simulink model "im_kalman_xy"  (R2025a)
settings: Solver=daessc  StartTime=0.0  StopTime=simlength  MaxStep=Tc  RelTol=Tc
undefined symbols (not defined in the file): Ad, Bd, C, cp, Ibez, Im, Inom, J, ki_inv_d, kp_inv_d, Lm, Qkalman, Rkalman, start_load, Tc, Ts, Vdc, w0
libraries: nesl_utility x11, fl_lib x6, simulink x2, im_lib x1
settings Model: SimulationMode=accelerator  Creator=dbagn  LastModifiedBy=dbagn
settings SolverCC: AlgebraicLoopSolver=TrustRegion
settings DataIOCC: ReturnWorkspaceOutputs=off
settings DebuggingCC: UnconnectedInputMsg=warning  UnconnectedOutputMsg=warning  UnconnectedLineMsg=warning
settings ModelReferenceCC: EnableRefExpFcnMdlSchedulingChecks=on
settings RTWCC: GPUComputeCapability=3.5  DLArmComputeVersion=19.05

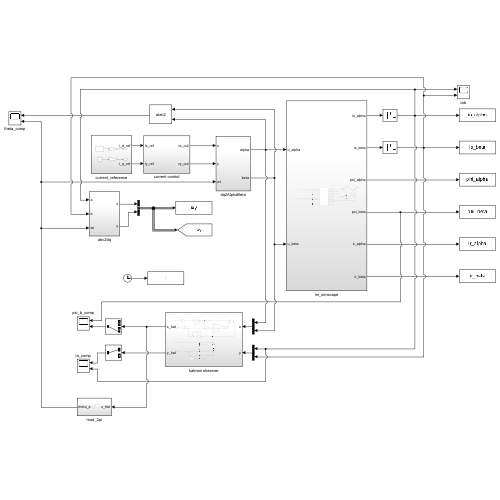
[thumbnail: Simulink's stored preview of the top-level diagram]
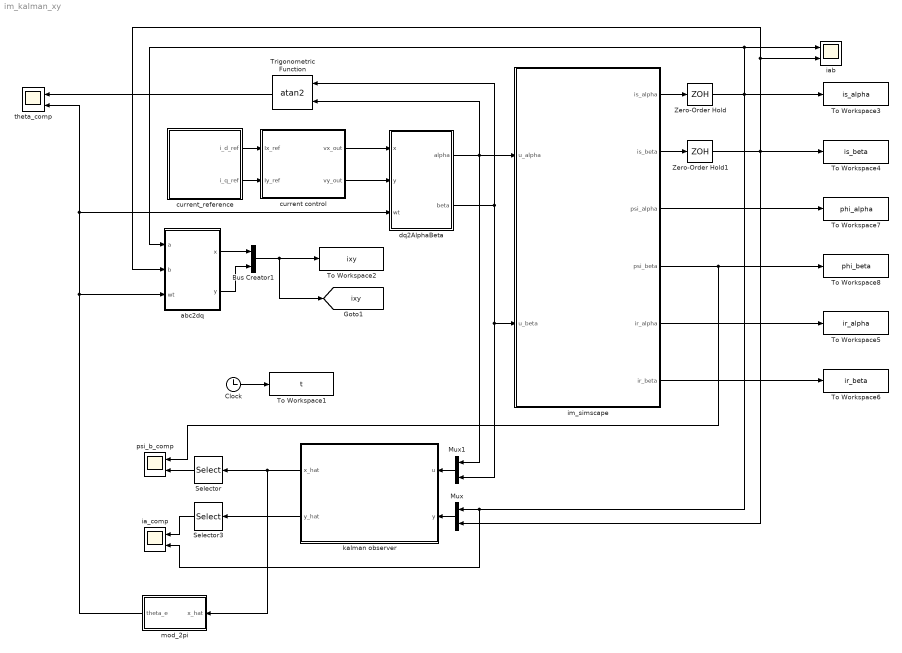
== system im_kalman_xy ==
  Bus Creator1 : BusCreator  Inputs=2
  Clock : Clock
  Mux : Mux  Inputs=2
  Mux1 : Mux  Inputs=2
  Selector : Selector  InputPortWidth=4  IndexOptions=Index vector (dialog)  Indices=4  OutputSizes=1
  Selector3 : Selector  InputPortWidth=2  IndexOptions=Index vector (dialog)  Indices=1  OutputSizes=1
  To Workspace1 : ToWorkspace  VariableName=t  SampleTime=Tc
      settings: MaxDataPoints=Nc
  To Workspace2 : ToWorkspace  VariableName=ixy  SampleTime=Tc
      settings: MaxDataPoints=Nc
  To Workspace3 : ToWorkspace  VariableName=is_alpha  SampleTime=Tc
      settings: MaxDataPoints=Nc
  To Workspace4 : ToWorkspace  VariableName=is_beta  SampleTime=Tc
      settings: MaxDataPoints=Nc
  To Workspace5 : ToWorkspace  VariableName=ir_alpha  SampleTime=Tc
      settings: MaxDataPoints=Nc
  To Workspace6 : ToWorkspace  VariableName=ir_beta  SampleTime=Tc
      settings: MaxDataPoints=Nc
  To Workspace7 : ToWorkspace  VariableName=phi_alpha  SampleTime=Tc
      settings: MaxDataPoints=Nc
  To Workspace8 : ToWorkspace  VariableName=phi_beta  SampleTime=Tc
      settings: MaxDataPoints=Nc
  Trigonometric Function : Trigonometry  Operator=atan2
  Zero-Order Hold : ZeroOrderHold  SampleTime=Ts
  Zero-Order Hold1 : ZeroOrderHold  SampleTime=Ts
  abc2dq : Subsystem
  current control : Subsystem
  current_reference : Subsystem
  dq2AlphaBeta : Subsystem
  ia_comp : Scope  NumInputPorts=2
      settings: ActiveDisplayYMinimum=-1099.3046905610083  ActiveDisplayYMaximum=2745.620661883479  DataLoggingVariableName=ScopeData3
  iab : Scope  NumInputPorts=2
      settings: ActiveDisplayYMinimum=-896.39173  ActiveDisplayYMaximum=667.17944
  im_simscape : Subsystem
  kalman observer : Subsystem
  mod_2pi : Subsystem
  psi_b_comp : Scope  NumInputPorts=2
      settings: ActiveDisplayYMinimum=-1.84097  ActiveDisplayYMaximum=1.77789  DataLoggingVariableName=ScopeData2
  theta_comp : Scope  NumInputPorts=2
      settings: ActiveDisplayYMinimum=-3.92689  ActiveDisplayYMaximum=3.92642
  tag scope: ixy=global
  wires:
  im_simscape/4(psi_beta) -> psi_b_comp/1, To Workspace8/1
  im_simscape/2(is_beta) -> Zero-Order Hold1/1
  im_simscape/1(is_alpha) -> Zero-Order Hold/1
  Mux1/1 -> kalman observer/1(u)
  Zero-Order Hold/1 -> Mux/1, ia_comp/2, To Workspace3/1, iab/1, abc2dq/1(a)
  Zero-Order Hold1/1 -> Mux/2, To Workspace4/1, abc2dq/2(b), iab/2
  Mux/1 -> kalman observer/2(y)
  Selector/1 -> psi_b_comp/2
  Selector3/1 -> ia_comp/1
  kalman observer/2(y_hat) -> Selector3/1
  current_reference/2(i_q_ref) -> current control/2(Iy_ref)
  current_reference/1(i_d_ref) -> current control/1(Ix_ref)
  Bus Creator1/1 -> To Workspace2/1, [ixy]
  abc2dq/2(y) -> Bus Creator1/2
  abc2dq/1(x) -> Bus Creator1/1
  current control/1(vx_out) -> dq2AlphaBeta/1(x)
  current control/2(vy_out) -> dq2AlphaBeta/2(y)
  dq2AlphaBeta/1(alpha) -> Trigonometric Function/2, Mux1/1, im_simscape/1(u_alpha)
  dq2AlphaBeta/2(beta) -> Mux1/2, im_simscape/2(u_beta), Trigonometric Function/1
  mod_2pi/1(theta_e) -> theta_comp/2, dq2AlphaBeta/3(wt), abc2dq/3(wt)
  Clock/1 -> To Workspace1/1
  kalman observer/1(x_hat) -> mod_2pi/1(x_hat), Selector/1
  im_simscape/3(psi_alpha) -> To Workspace7/1
  im_simscape/5(ir_alpha) -> To Workspace5/1
  im_simscape/6(ir_beta) -> To Workspace6/1
  Trigonometric Function/1 -> theta_comp/1

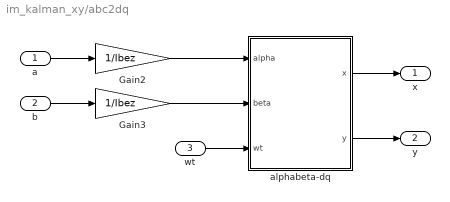
== system im_kalman_xy/abc2dq ==
  a : Inport
  b : Inport  Port=2
  wt : Inport  Port=3
  Gain2 : Gain  Gain=1/Ibez
  Gain3 : Gain  Gain=1/Ibez
  alphabeta-dq : Subsystem
  x : Outport  VectorParamsAs1DForOutWhenUnconnected=off
  y : Outport  Port=2  VectorParamsAs1DForOutWhenUnconnected=off
  wires:
  a/1 -> Gain2/1
  b/1 -> Gain3/1
  wt/1 -> alphabeta-dq/3(wt)
  alphabeta-dq/1(x) -> x/1
  alphabeta-dq/2(y) -> y/1
  Gain2/1 -> alphabeta-dq/1(alpha)
  Gain3/1 -> alphabeta-dq/2(beta)

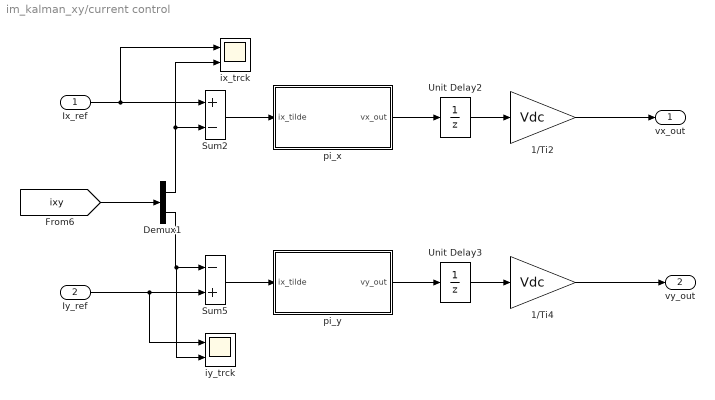
== system im_kalman_xy/current control ==
  Ix_ref : Inport
  Iy_ref : Inport  Port=2
  1/Ti2 : Gain  Gain=Vdc  SaturateOnIntegerOverflow=on  OutDataTypeStr=Inherit: Same as input  ParamDataTypeStr=Inherit: Same as input
  1/Ti4 : Gain  Gain=Vdc  SaturateOnIntegerOverflow=on  OutDataTypeStr=Inherit: Same as input  ParamDataTypeStr=Inherit: Same as input
  Demux1 : Demux  Outputs=2
  Sum2 : Sum  Inputs=+-  SaturateOnIntegerOverflow=on
  Sum5 : Sum  Inputs=-+  SaturateOnIntegerOverflow=on
  Unit Delay2 : UnitDelay  SampleTime=Ts  HasFrameUpgradeWarning=on
  Unit Delay3 : UnitDelay  SampleTime=Ts  HasFrameUpgradeWarning=on
  ix_trck : Scope  NumInputPorts=2
      settings: ActiveDisplayYMinimum=0.20638  ActiveDisplayYMaximum=0.72674
  iy_trck : Scope  NumInputPorts=2
      settings: ActiveDisplayYMinimum=-0.16299  ActiveDisplayYMaximum=1.1565  DataLoggingVariableName=ScopeData2
  pi_x : Subsystem
  pi_y : Subsystem
  vx_out : Outport  VectorParamsAs1DForOutWhenUnconnected=off
  vy_out : Outport  Port=2  VectorParamsAs1DForOutWhenUnconnected=off
  wires:
  Iy_ref/1 -> iy_trck/1, Sum5/2
  Unit Delay3/1 -> 1/Ti4/1
  Unit Delay2/1 -> 1/Ti2/1
  [ixy] -> Demux1/1
  Demux1/2 -> iy_trck/2, Sum5/1
  Ix_ref/1 -> ix_trck/1, Sum2/1
  Demux1/1 -> ix_trck/2, Sum2/2
  pi_x/1(vx_out) -> Unit Delay2/1
  pi_y/1(vy_out) -> Unit Delay3/1
  Sum5/1 -> pi_y/1(ix_tilde)
  Sum2/1 -> pi_x/1(ix_tilde)
  1/Ti2/1 -> vx_out/1
  1/Ti4/1 -> vy_out/1

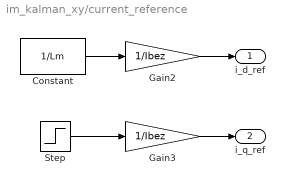
== system im_kalman_xy/current_reference ==
  Constant : Constant  Value=1/Lm
  Gain2 : Gain  Gain=1/Ibez
  Gain3 : Gain  Gain=1/Ibez
  Step : Step  Time=start_load  After=sqrt(Inom^2-Im^2)*sqrt(2)  SampleTime=0
  i_d_ref : Outport
  i_q_ref : Outport  Port=2
  wires:
  Step/1 -> Gain3/1
  Constant/1 -> Gain2/1
  Gain2/1 -> i_d_ref/1
  Gain3/1 -> i_q_ref/1

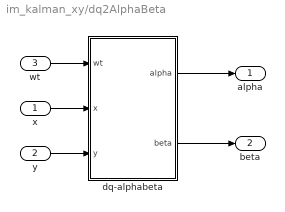
== system im_kalman_xy/dq2AlphaBeta ==
  x : Inport
  y : Inport  Port=2
  wt : Inport  Port=3
  dq-alphabeta : Subsystem
  alpha : Outport  VectorParamsAs1DForOutWhenUnconnected=off
  beta : Outport  Port=2  VectorParamsAs1DForOutWhenUnconnected=off
  wires:
  x/1 -> dq-alphabeta/2(x)
  y/1 -> dq-alphabeta/3(y)
  wt/1 -> dq-alphabeta/1(wt)
  dq-alphabeta/1(alpha) -> alpha/1
  dq-alphabeta/2(beta) -> beta/1

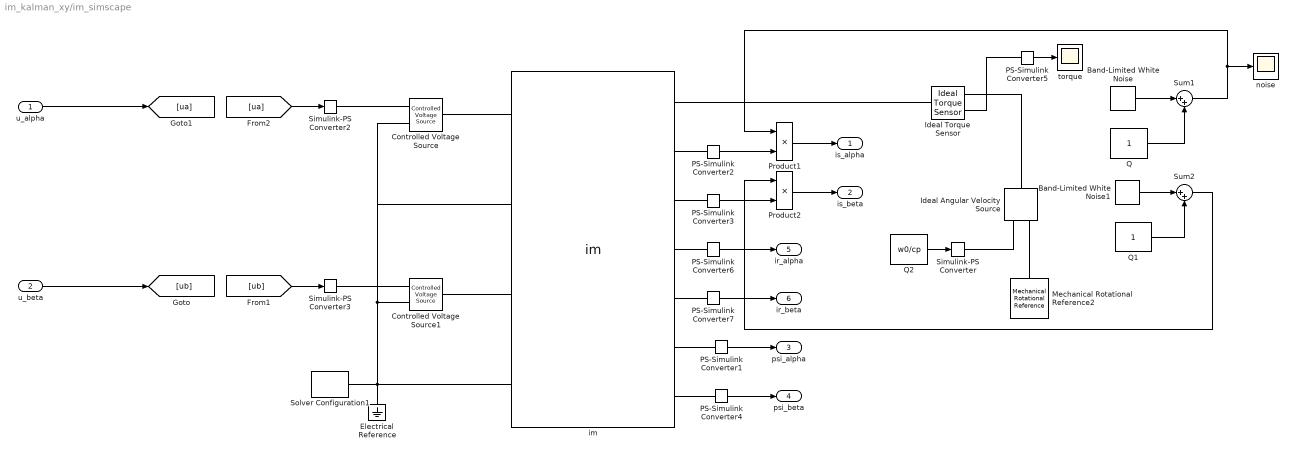
== system im_kalman_xy/im_simscape ==
  u_alpha : Inport
  u_beta : Inport  Port=2
  Band-Limited White Noise : simulink/Sources/Band-Limited White Noise  Cov=2e-10  Ts=Tc  seed=[23341]
  Band-Limited White Noise1 : simulink/Sources/Band-Limited White Noise  Cov=2e-10  Ts=Tc  seed=[23341]
  Controlled Voltage Source : fl_lib/Electrical/Electrical Sources/Controlled Voltage Source
  Controlled Voltage Source1 : fl_lib/Electrical/Electrical Sources/Controlled Voltage Source
  Electrical Reference : fl_lib/Electrical/Electrical Elements/Electrical Reference
  Ideal Angular Velocity Source : fl_lib/Mechanical/Mechanical Sources/Ideal Angular Velocity Source
  Ideal Torque Sensor : fl_lib/Mechanical/Mechanical Sensors/Ideal Torque Sensor
  Mechanical Rotational Reference2 : fl_lib/Mechanical/Rotational Elements/Mechanical Rotational Reference
  PS-Simulink Converter{1..7} (7 alike) : nesl_utility/PS-Simulink Converter  PhysicalDomain=network_engine_domain  SubClassName=ps_output  LeftPortType=input  RightPortType=output  PseudoPeriodic=off  Frequencies=[]  VectorFormat=1-D array  Unit=1  AffineConversion=off
  Product1 : Product
  Product2 : Product
  Q : Constant
  Q1 : Constant
  Q2 : Constant  Value=w0/cp
  Simulink-PS Converter : nesl_utility/Simulink-PS Converter  PhysicalDomain=network_engine_domain  SubClassName=ps_input  LeftPortType=input  RightPortType=output  PseudoPeriodic=off  Frequencies=[]  NoiseDistribution=none  NoiseParameters=[]  Unit=1  AffineConversion=off  FilteringAndDerivatives=provide  SimscapeFilterOrder=1  InputFilterTimeConstant=0.001  UdotUserProvided=0
  Simulink-PS Converter2 : nesl_utility/Simulink-PS Converter  PhysicalDomain=network_engine_domain  SubClassName=ps_input  LeftPortType=input  RightPortType=output  PseudoPeriodic=off  Frequencies=[]  NoiseDistribution=none  NoiseParameters=[]  Unit=1  AffineConversion=off  FilteringAndDerivatives=provide  SimscapeFilterOrder=1  InputFilterTimeConstant=0.001  UdotUserProvided=0
  Simulink-PS Converter3 : nesl_utility/Simulink-PS Converter  PhysicalDomain=network_engine_domain  SubClassName=ps_input  LeftPortType=input  RightPortType=output  PseudoPeriodic=off  Frequencies=[]  NoiseDistribution=none  NoiseParameters=[]  Unit=1  AffineConversion=off  FilteringAndDerivatives=provide  SimscapeFilterOrder=1  InputFilterTimeConstant=0.001  UdotUserProvided=0
  Solver Configuration1 : nesl_utility/Solver Configuration  PhysicalDomain=network_engine_domain  SubClassName=solver  LeftPortType=input  RightPortType=generic  Tones=[]  Harmonics=[]  SimulateNoise=off  Profile=off  UseLocalSampling=off  EnableSwitchedLinearOptims=on  FrequencyDomain=off  UseCCode=off  RelTol=0.001  AbsTol=1e-06  MinStep=1e-09  ToWorkspace=off  RevertToSquareIcSolve=off  NumHomotopyIterations=100  PhasorMode=off  PhasorModeNumHarmonics=1  ConsistencySolver=NEWTON_FTOL  IndexReductionMethod=DerivativeReplacement  DoDC=off  ResidualTolerance=1e-09  ConsistencyTolSource=GLOBAL  ConsistencyAbsTol=0.001  ConsistencyRelTol=0.001  ConsistencyTolFactor=0.001  UseLocalSolver=off  LocalSolverChoice=NE_TRAPEZOIDAL_ADVANCER  ResolveIndetEquations=on  FunctionEvalNumThread=1  LocalSolverSampleTime=Tc  DoFixedCost=off  MaxNonlinIter=3  MaxModeIter=2  ComputeImpulses=off  ImpulseIterations=2  LinearAlgebra=auto  LinearAlgebraNumThread=0  EquationFormulation=NE_TIME_EF  DelaysMemoryBudget=1024  AutomaticFiltering=on  FilteringTimeConstant=0.001  PartitionStorageMethod=AS_NEEDED  PartitionMemoryBudget=1024  PartitionMethod=ROBUST  MultibodyUseLocalSolver=off  MultibodyLocalSolverChoice=ODE1  MultibodyLocalSolverSampleTime=0.001
  Sum1 : Sum  Inputs=|++
  Sum2 : Sum  Inputs=|++
  im : im_lib/im  Lm=Lm H  Rs=Rs Ohm  Lr=Lr H  Ls=Ls H  Rr=Rr Ohm  J=J kg*m^2  cp=cp
      settings: InternalSimscapePortConfiguration="{\"Bottom\":[],\"Left\":[{\"id\":\"u_alpha_p\",\"label\":\"u_alpha+\",\"type\":\"foundation.electrical.electrical\"},{\"id\":\"u_alpha_n\",\"label\":\"u_alpha-\",\"type\":\"foundation.electrical.electrical\"},{\"id\":\"u_beta_p\",\"label\":\"u_beta+\",\"type\":\"foundation.electrical.electrical\"},{\"id\":\"u_beta_n\",\"label\":\"u_beta-\",\"type\":\"foundation.electrical.electrical\"}],\"Right\":[{\"id\":\"S\",\"label\":\"S\",\"type\":\"foundation.mechanical.rotational.rotational\"},{\"id\":\"is_alpha\",\"label\":\"is_alpha\",\"type\":\"output\"},{\"id\":\"is_beta\",\"label\":\"is_beta\",\"type\":\"output\"},{\"id\":\"ir_alpha\",\"label\":\"ir_alpha\",\"type\":\"output\"},{\"id\":\"ir_beta\",\"label\":\"ir_beta\",\"type\":\"output\"},{\"id\":\"psi_alpha\",\"label\":\"psi_alpha\",\"type\":\"output\"},{\"id\":\"psi_beta\",\"label\":\"psi_beta\",\"type\":\"output\"}],\"Top\":[]}"
  noise : Scope
      settings: ActiveDisplayYMinimum=0.87016  ActiveDisplayYMaximum=1.17211  DataLoggingVariableName=ScopeData3
  torque : Scope
      settings: ActiveDisplayYMinimum=-225649.75684  ActiveDisplayYMaximum=27994.54384
  is_alpha : Outport
  is_beta : Outport  Port=2
  psi_alpha : Outport  Port=3
  psi_beta : Outport  Port=4
  ir_alpha : Outport  Port=5
  ir_beta : Outport  Port=6
  wires:
  u_alpha/1 -> [ua]
  [ua] -> Simulink-PS Converter2/1
  u_beta/1 -> [ub]
  [ub] -> Simulink-PS Converter3/1
  PS-Simulink Converter1/1 -> psi_alpha/1
  PS-Simulink Converter4/1 -> psi_beta/1
  Q/1 -> Sum1/2
  PS-Simulink Converter2/1 -> Product1/2
  Product1/1 -> is_alpha/1
  PS-Simulink Converter3/1 -> Product2/2
  Product2/1 -> is_beta/1
  Q1/1 -> Sum2/2
  Sum2/1 -> Product2/1
  Q2/1 -> Simulink-PS Converter/1
  PS-Simulink Converter5/1 -> torque/1
  Sum1/1 -> Product1/1, noise/1
  Band-Limited White Noise/1 -> Sum1/1
  Band-Limited White Noise1/1 -> Sum2/1
  PS-Simulink Converter6/1 -> ir_alpha/1
  PS-Simulink Converter7/1 -> ir_beta/1
  connections:
  Controlled Voltage Source/RConn1 -- Simulink-PS Converter2/RConn1
  Simulink-PS Converter3/RConn1 -- Controlled Voltage Source1/RConn1
  im/RConn2 -- PS-Simulink Converter2/LConn1
  im/RConn3 -- PS-Simulink Converter3/LConn1
  Ideal Angular Velocity Source/RConn2 -- Mechanical Rotational Reference2/LConn1
  Simulink-PS Converter/RConn1 -- Ideal Angular Velocity Source/RConn1
  Ideal Torque Sensor/LConn1 -- im/RConn1
  Ideal Torque Sensor/RConn1 -- Ideal Angular Velocity Source/LConn1
  Ideal Torque Sensor/RConn2 -- PS-Simulink Converter5/LConn1
  Controlled Voltage Source1/RConn2 -- Controlled Voltage Source/RConn2 -- im/LConn2 -- Electrical Reference/LConn1 -- im/LConn4 -- Solver Configuration1/RConn1
  im/LConn3 -- Controlled Voltage Source1/LConn1
  Controlled Voltage Source/LConn1 -- im/LConn1
  im/RConn6 -- PS-Simulink Converter1/LConn1
  im/RConn7 -- PS-Simulink Converter4/LConn1
  im/RConn4 -- PS-Simulink Converter6/LConn1
  im/RConn5 -- PS-Simulink Converter7/LConn1

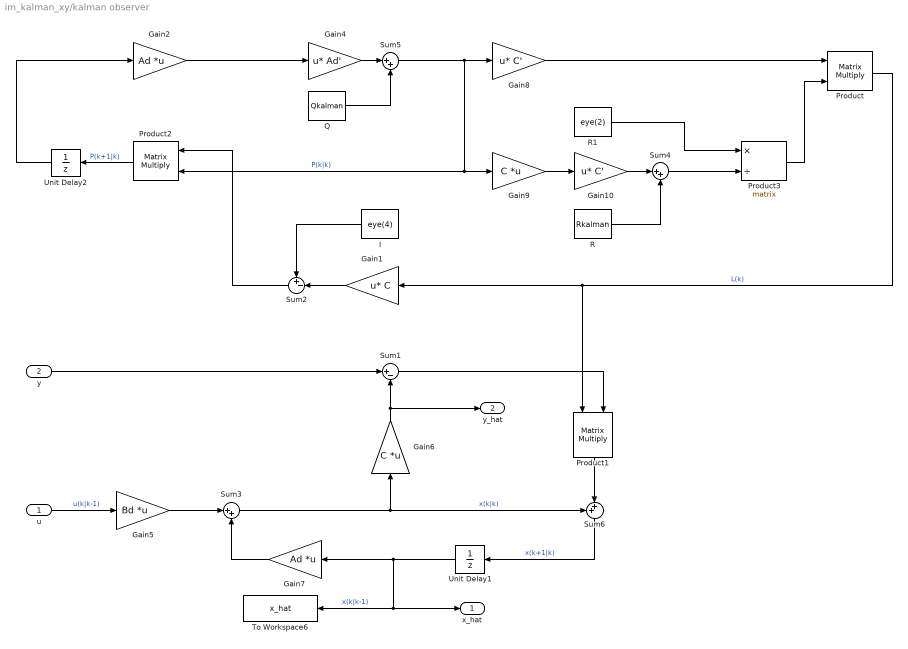
== system im_kalman_xy/kalman observer ==
  u : Inport
  y : Inport  Port=2
  Gain1 : Gain  Gain=C  Multiplication=Matrix(u*K)
  Gain10 : Gain  Gain=C'  Multiplication=Matrix(u*K)
  Gain2 : Gain  Gain=Ad  Multiplication=Matrix(K*u)
  Gain4 : Gain  Gain=Ad'  Multiplication=Matrix(u*K)
  Gain5 : Gain  Gain=Bd  Multiplication=Matrix(K*u)
  Gain6 : Gain  Gain=C  Multiplication=Matrix(K*u)
  Gain7 : Gain  Gain=Ad  Multiplication=Matrix(K*u)
  Gain8 : Gain  Gain=C'  Multiplication=Matrix(u*K)
  Gain9 : Gain  Gain=C  Multiplication=Matrix(K*u)
  I : Constant  Value=eye(4)
  Product : Product  Multiplication=Matrix(*)
  Product1 : Product  Multiplication=Matrix(*)
  Product2 : Product  Multiplication=Matrix(*)
  Product3 : Product  Inputs=*/  Multiplication=Matrix(*)
  Q : Constant  Value=Qkalman
  R : Constant  Value=Rkalman
  R1 : Constant  Value=eye(2)
  Sum1 : Sum  Inputs=|+-
  Sum2 : Sum  Inputs=+-|
  Sum3 : Sum  Inputs=|++
  Sum4 : Sum  Inputs=|++
  Sum5 : Sum  Inputs=|++
  Sum6 : Sum  Inputs=++|
  To Workspace6 : ToWorkspace  VariableName=x_hat  SampleTime=Tc
      settings: MaxDataPoints=Nc
  Unit Delay1 : UnitDelay  InitialCondition=[0 0 1 0]  SampleTime=Ts  HasFrameUpgradeWarning=on
  Unit Delay2 : UnitDelay  InitialCondition=Qkalman  SampleTime=Ts  HasFrameUpgradeWarning=on
  x_hat : Outport
  y_hat : Outport  Port=2
  wires:
  Gain5/1 -> Sum3/1
  Gain7/1 -> Sum3/2
  Gain6/1 -> Sum1/2, y_hat/1
  Sum5/1 -> Product2/2, Gain9/1, Gain8/1  "P(k|k)"
  Gain2/1 -> Gain4/1
  Gain4/1 -> Sum5/1
  Q/1 -> Sum5/2
  Gain9/1 -> Gain10/1
  R/1 -> Sum4/2
  Gain10/1 -> Sum4/1
  Gain8/1 -> Product/1
  Product/1 -> Gain1/1, Product1/1  "L(k)"
  Product2/1 -> Unit Delay2/1  "P(k+1|k)"
  Sum2/1 -> Product2/1
  Unit Delay2/1 -> Gain2/1
  Sum6/1 -> Unit Delay1/1  "x(k+1|k)"
  I/1 -> Sum2/1
  Gain1/1 -> Sum2/2
  Sum1/1 -> Product1/2
  y/1 -> Sum1/1
  Sum4/1 -> Product3/2
  Product3/1 -> Product/2
  R1/1 -> Product3/1
  Product1/1 -> Sum6/2
  u/1 -> Gain5/1  "u(k|k-1)"
  Sum3/1 -> Gain6/1, Sum6/1  "x(k|k)"
  Unit Delay1/1 -> To Workspace6/1, x_hat/1, Gain7/1  "x(k|k-1)"

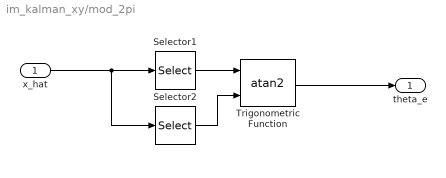
== system im_kalman_xy/mod_2pi ==
  x_hat : Inport
  Selector1 : Selector  InputPortWidth=4  IndexOptions=Index vector (dialog)  Indices=4  OutputSizes=1
  Selector2 : Selector  InputPortWidth=4  IndexOptions=Index vector (dialog)  Indices=3  OutputSizes=1
  Trigonometric Function : Trigonometry  Operator=atan2
  theta_e : Outport
  wires:
  Trigonometric Function/1 -> theta_e/1
  Selector1/1 -> Trigonometric Function/1
  Selector2/1 -> Trigonometric Function/2
  x_hat/1 -> Selector2/1, Selector1/1

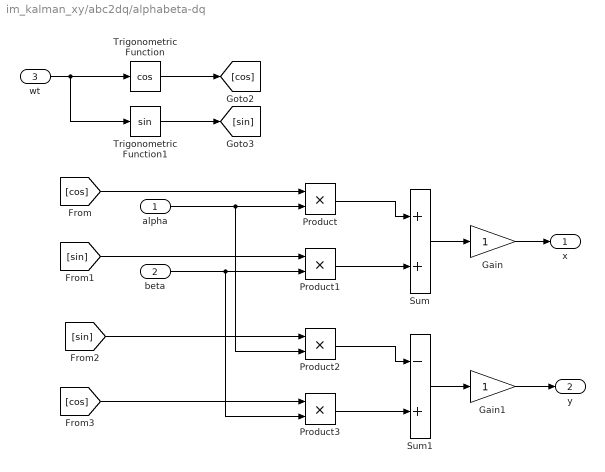
== system im_kalman_xy/abc2dq/alphabeta-dq ==
  alpha : Inport
  beta : Inport  Port=2
  wt : Inport  Port=3
  Gain : Gain
  Gain1 : Gain
  Product{,1..3} (4 alike) : Product  RndMeth=Zero
  Sum : Sum
  Sum1 : Sum  Inputs=-+
  Trigonometric Function : Trigonometry  Operator=cos
  Trigonometric Function1 : Trigonometry
  x : Outport  VectorParamsAs1DForOutWhenUnconnected=off
  y : Outport  Port=2  VectorParamsAs1DForOutWhenUnconnected=off
  wires:
  [cos] -> Product/1
  alpha/1 -> Product/2, Product2/2
  Product/1 -> Sum/1
  Product1/1 -> Sum/2
  [sin] -> Product1/1
  beta/1 -> Product1/2, Product3/2
  Sum/1 -> Gain/1
  [sin] -> Product2/1
  Product2/1 -> Sum1/1
  Product3/1 -> Sum1/2
  [cos] -> Product3/1
  Sum1/1 -> Gain1/1
  Gain/1 -> x/1
  Gain1/1 -> y/1
  Trigonometric Function1/1 -> [sin]
  Trigonometric Function/1 -> [cos]
  wt/1 -> Trigonometric Function/1, Trigonometric Function1/1

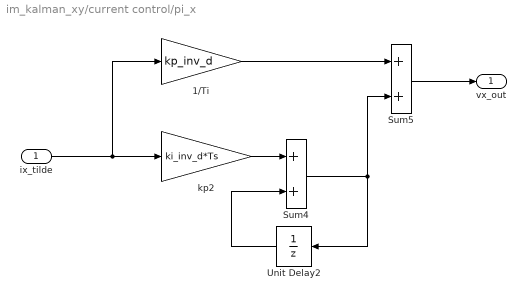
== system im_kalman_xy/current control/pi_x ==
  ix_tilde : Inport
  1/Ti : Gain  Gain=kp_inv_d  SaturateOnIntegerOverflow=on  OutDataTypeStr=Inherit: Same as input  ParamDataTypeStr=Inherit: Same as input
  Sum4 : Sum  SaturateOnIntegerOverflow=on
  Sum5 : Sum  SaturateOnIntegerOverflow=on
  Unit Delay2 : UnitDelay  SampleTime=Ts  HasFrameUpgradeWarning=on
  kp2 : Gain  Gain=ki_inv_d*Ts  SaturateOnIntegerOverflow=on  OutDataTypeStr=Inherit: Same as input  ParamDataTypeStr=Inherit: Same as input
  vx_out : Outport  VectorParamsAs1DForOutWhenUnconnected=off
  wires:
  ix_tilde/1 -> kp2/1, 1/Ti/1
  Sum5/1 -> vx_out/1
  Sum4/1 -> Unit Delay2/1, Sum5/2
  Unit Delay2/1 -> Sum4/2
  1/Ti/1 -> Sum5/1
  kp2/1 -> Sum4/1

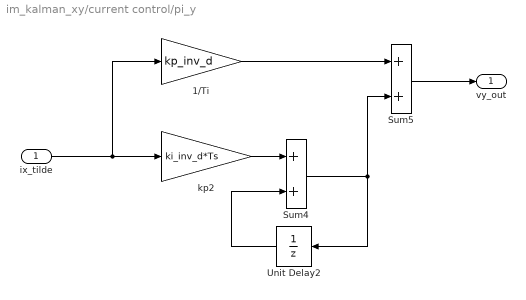
== system im_kalman_xy/current control/pi_y ==
  ix_tilde : Inport
  1/Ti : Gain  Gain=kp_inv_d  SaturateOnIntegerOverflow=on  OutDataTypeStr=Inherit: Same as input  ParamDataTypeStr=Inherit: Same as input
  Sum4 : Sum  SaturateOnIntegerOverflow=on
  Sum5 : Sum  SaturateOnIntegerOverflow=on
  Unit Delay2 : UnitDelay  SampleTime=Ts  HasFrameUpgradeWarning=on
  kp2 : Gain  Gain=ki_inv_d*Ts  SaturateOnIntegerOverflow=on  OutDataTypeStr=Inherit: Same as input  ParamDataTypeStr=Inherit: Same as input
  vy_out : Outport  VectorParamsAs1DForOutWhenUnconnected=off
  wires:
  kp2/1 -> Sum4/1
  1/Ti/1 -> Sum5/1
  Unit Delay2/1 -> Sum4/2
  Sum4/1 -> Sum5/2, Unit Delay2/1
  Sum5/1 -> vy_out/1
  ix_tilde/1 -> 1/Ti/1, kp2/1

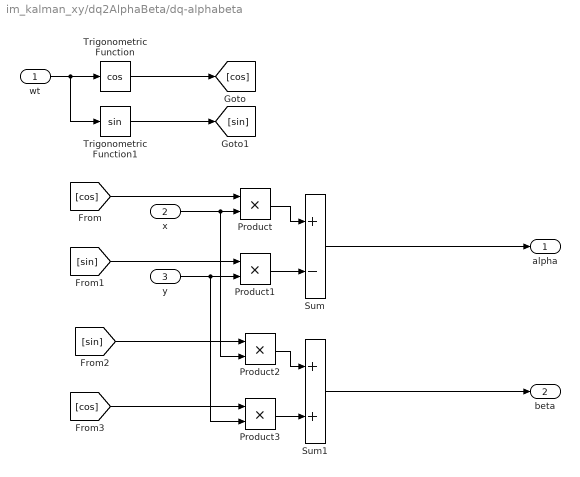
== system im_kalman_xy/dq2AlphaBeta/dq-alphabeta ==
  wt : Inport
  x : Inport  Port=2
  y : Inport  Port=3
  Product{,1..3} (4 alike) : Product  RndMeth=Zero
  Sum : Sum  Inputs=+-
  Sum1 : Sum
  Trigonometric Function : Trigonometry  Operator=cos
  Trigonometric Function1 : Trigonometry
  alpha : Outport  VectorParamsAs1DForOutWhenUnconnected=off
  beta : Outport  Port=2  VectorParamsAs1DForOutWhenUnconnected=off
  wires:
  Sum1/1 -> beta/1
  [cos] -> Product3/1
  Product3/1 -> Sum1/2
  Product2/1 -> Sum1/1
  [sin] -> Product2/1
  Sum/1 -> alpha/1
  y/1 -> Product3/2, Product1/2
  [sin] -> Product1/1
  Product1/1 -> Sum/2
  Product/1 -> Sum/1
  x/1 -> Product2/2, Product/2
  [cos] -> Product/1
  Trigonometric Function1/1 -> [sin]
  Trigonometric Function/1 -> [cos]
  wt/1 -> Trigonometric Function/1, Trigonometric Function1/1
